simulink model "uz_ssi_interface_2023a"  (R2023a)
settings: Solver=FixedStepDiscrete  StartTime=0.0  StopTime=0.003  RelTol=1e-3
values from neighbouring files (symbols this model uses):
  binary_or_gray = false    [uz_ssi_interface_init.m]
  bit_sum = ssi_encoder_bit_width_multi_turn+ssi_encoder_bit_width_single_turn+ssi_encoder_number_of_status_bits    [uz_ssi_interface_init.m]
  delay_first_clk_on_off = true    [uz_ssi_interface_init.m]
  f_ADC = 10e3    (= 10000)    [uz_ssi_interface_init.m]
  f_clock = 100e6    (= 100000000)    [uz_ssi_interface_init.m]
  ssi_clk_divider = 25    [uz_ssi_interface_init.m]
  ssi_encoder_bit_width_multi_turn = uint32(0)    [uz_ssi_interface_init.m]
  ssi_encoder_bit_width_single_turn = uint32(14)    [uz_ssi_interface_init.m]
  ssi_encoder_number_of_status_bits = uint32(0)    [uz_ssi_interface_init.m]
  t_ADC = 1/f_ADC    (= 0.0001)    [uz_ssi_interface_init.m]
  t_clock = 1/f_clock    (= 1e-08)    [uz_ssi_interface_init.m]
undefined symbols (not defined in the file or in its folder): PLL
libraries: hdlsllib x42, simulink x14, simulink_extras x5, spsSampleandHoldLib x1
(part 2 of 2)

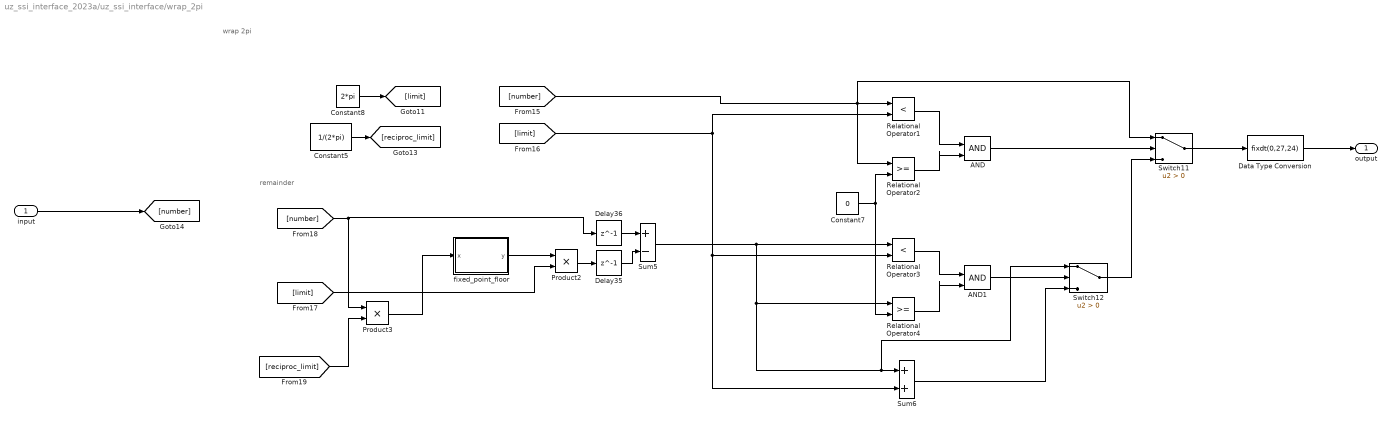
== system uz_ssi_interface_2023a/uz_ssi_interface/wrap_2pi ==
  note: wrap 2pi
  note: remainder
  input : Inport
  AND : Logic  IconShape=distinctive  AllPortsSameDT=off  OutDataTypeStr=boolean
  AND1 : Logic  IconShape=distinctive  AllPortsSameDT=off  OutDataTypeStr=boolean
  Constant5 : Constant  Value=1/(2*pi)  OutDataTypeStr=fixdt(0,18,20)  SampleTime=-1
  Constant7 : Constant  Value=0  OutDataTypeStr=fixdt(0,27,24)  SampleTime=-1
  Constant8 : Constant  Value=2*pi  OutDataTypeStr=fixdt(0,18,15)  SampleTime=-1
  Data Type Conversion : DataTypeConversion  OutDataTypeStr=fixdt(0,27,24)  SaturateOnIntegerOverflow=off  RndMeth=Floor
  Delay35 : Delay  DelayLength=1  InitialCondition=0
  Delay36 : Delay  DelayLength=1  InitialCondition=0
  Product2 : Product  OutDataTypeStr=fixdt(0,27,24)
  Product3 : Product  OutDataTypeStr=fixdt(0,27,24)
  Relational Operator1 : RelationalOperator  Operator=<  OutDataTypeStr=boolean  RndMeth=Simplest  InputSameDT=off
  Relational Operator2 : RelationalOperator  OutDataTypeStr=boolean  RndMeth=Simplest  InputSameDT=off
  Relational Operator3 : RelationalOperator  Operator=<  OutDataTypeStr=boolean  RndMeth=Simplest  InputSameDT=off
  Relational Operator4 : RelationalOperator  OutDataTypeStr=boolean  RndMeth=Simplest  InputSameDT=off
  Sum5 : Sum  Inputs=+-  OutDataTypeStr=fixdt(0,27,24)
  Sum6 : Sum  OutDataTypeStr=fixdt(0,27,24)
  Switch11 : Switch  Criteria=u2 > Threshold  SaturateOnIntegerOverflow=off  InputSameDT=off
  Switch12 : Switch  Criteria=u2 > Threshold  SaturateOnIntegerOverflow=off  InputSameDT=off
  fixed_point_floor : MATLAB Function  TreatAsAtomicUnit=on
  output : Outport
  wires:
  [number] -> Relational Operator2/1, Switch11/1, Relational Operator1/1
  Product2/1 -> Delay35/1
  [number] -> Delay36/1, Product3/1
  [reciproc_limit] -> Product3/2
  Delay35/1 -> Sum5/2
  Switch11/1 -> Data Type Conversion/1
  Relational Operator2/1 -> AND/2
  AND/1 -> Switch11/2
  Sum5/1 -> Switch12/1, Sum6/1, Relational Operator4/1, Relational Operator3/1
  Relational Operator1/1 -> AND/1
  [limit] -> Relational Operator1/2, Sum6/2, Relational Operator3/2
  Sum6/1 -> Switch12/3
  Delay36/1 -> Sum5/1
  Constant7/1 -> Relational Operator2/2, Relational Operator4/2
  Constant5/1 -> [reciproc_limit]
  Relational Operator4/1 -> AND1/2
  fixed_point_floor/1(y) -> Product2/1
  Product3/1 -> fixed_point_floor/1(x)
  AND1/1 -> Switch12/2
  [limit] -> Product2/2
  input/1 -> [number]
  Relational Operator3/1 -> AND1/1
  Switch12/1 -> Switch11/3
  Constant8/1 -> [limit]
  Data Type Conversion/1 -> output/1

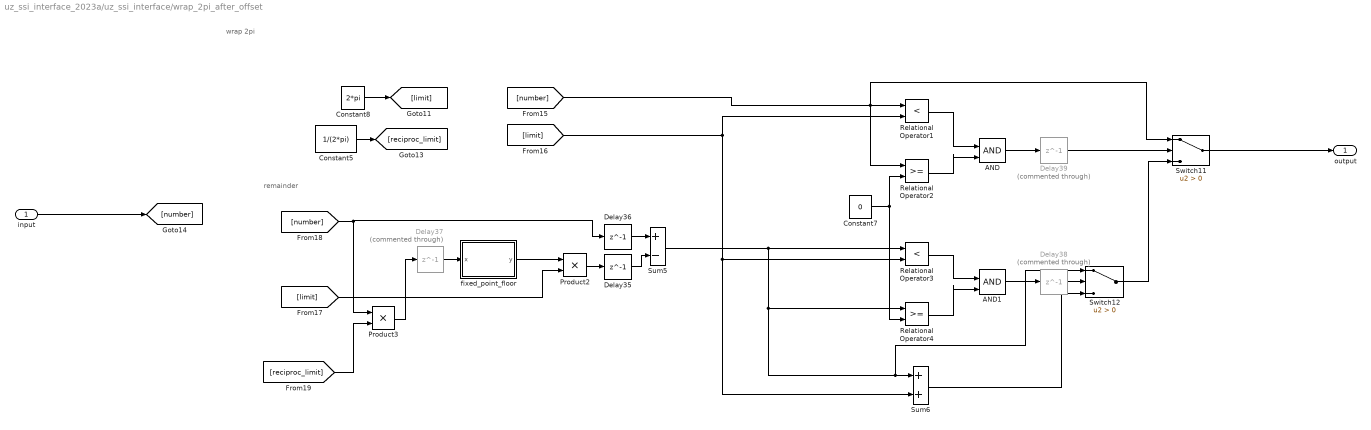
== system uz_ssi_interface_2023a/uz_ssi_interface/wrap_2pi_after_offset ==
  note: wrap 2pi
  note: remainder
  input : Inport
  AND : Logic  IconShape=distinctive  AllPortsSameDT=off  OutDataTypeStr=boolean
  AND1 : Logic  IconShape=distinctive  AllPortsSameDT=off  OutDataTypeStr=boolean
  Constant5 : Constant  Value=1/(2*pi)  OutDataTypeStr=fixdt(0,18,20)  SampleTime=-1
  Constant7 : Constant  Value=0  OutDataTypeStr=fixdt(0,27,24)  SampleTime=-1
  Constant8 : Constant  Value=2*pi  OutDataTypeStr=fixdt(0,18,15)  SampleTime=-1
  Delay35 : Delay  DelayLength=1  InitialCondition=0
  Delay36 : Delay  DelayLength=1  InitialCondition=0
  Delay37 : Delay  Commented=through  DelayLength=1  InitialCondition=0
  Delay38 : Delay  Commented=through  DelayLength=1
  Delay39 : Delay  Commented=through  DelayLength=1
  Product2 : Product  OutDataTypeStr=fixdt(0,27,24)
  Product3 : Product  OutDataTypeStr=fixdt(1,27,23)
  Relational Operator1 : RelationalOperator  Operator=<  OutDataTypeStr=boolean  RndMeth=Simplest  InputSameDT=off
  Relational Operator2 : RelationalOperator  OutDataTypeStr=boolean  RndMeth=Simplest  InputSameDT=off
  Relational Operator3 : RelationalOperator  Operator=<  OutDataTypeStr=boolean  RndMeth=Simplest  InputSameDT=off
  Relational Operator4 : RelationalOperator  OutDataTypeStr=boolean  RndMeth=Simplest  InputSameDT=off
  Sum5 : Sum  Inputs=+-  OutDataTypeStr=fixdt(0,27,24)
  Sum6 : Sum  OutDataTypeStr=fixdt(0,27,24)
  Switch11 : Switch  Criteria=u2 > Threshold  SaturateOnIntegerOverflow=off  InputSameDT=off
  Switch12 : Switch  Criteria=u2 > Threshold  SaturateOnIntegerOverflow=off  InputSameDT=off
  fixed_point_floor : MATLAB Function  TreatAsAtomicUnit=on
  output : Outport
  wires:
  [number] -> Relational Operator2/1, Switch11/1, Relational Operator1/1
  Product2/1 -> Delay35/1
  [number] -> Delay36/1, Product3/1
  [reciproc_limit] -> Product3/2
  Product3/1 -> Delay37/1
  Delay35/1 -> Sum5/2
  Switch11/1 -> output/1
  Relational Operator2/1 -> AND/2
  AND1/1 -> Delay38/1
  Delay39/1 -> Switch11/2
  Sum5/1 -> Switch12/1, Sum6/1, Relational Operator4/1, Relational Operator3/1
  Relational Operator1/1 -> AND/1
  [limit] -> Relational Operator1/2, Sum6/2, Relational Operator3/2
  AND/1 -> Delay39/1
  Sum6/1 -> Switch12/3
  Delay36/1 -> Sum5/1
  Constant7/1 -> Relational Operator2/2, Relational Operator4/2
  Constant5/1 -> [reciproc_limit]
  Relational Operator4/1 -> AND1/2
  fixed_point_floor/1(y) -> Product2/1
  Delay37/1 -> fixed_point_floor/1(x)
  Delay38/1 -> Switch12/2
  [limit] -> Product2/2
  input/1 -> [number]
  Relational Operator3/1 -> AND1/1
  Switch12/1 -> Switch11/3
  Constant8/1 -> [limit]

== matlab function uz_ssi_interface_2023a/uz_ssi_interface/sample_serial_ssi_data/sample_serial_data ==
  data: clk input; data_out output; data_in input; bit_width input; data_valid output
function [data_out, data_valid]  = sample_serial_data(clk, data_in, bit_width)
    % Function to sample serial data bits of configurable length
    % Inputs:
    %   - data_in: Single bit of serial data to be sampled (1 or 0)
    %   - clk: Input clock signal (high when data is to be sampled)
    %   - bit_width: Number of bits to be sampled (configurable length)
    %
    % Output:
    %   - data_out: Integer value of the concatenated data bits after sampling
    %   - data_valid: high when all bits have been sampled

    persistent data_buffer bit_count

    if isempty(data_buffer)
        % Initialize buffer as a fixed-point number with 64 bits and unsigned
        data_buffer = fi(0,0,64,0); 
        bit_count = uint32(bit_width); 
    end

    % Sample the data when the clock is high
    if clk == 1

        % Add the incoming bit to the data buffer
        data_buffer = bitset(data_buffer,bit_count,data_in);

        % Decrement the bit counter
        bit_count = bit_count - 1;
    end

    % When the required length is reached, output the data
    if bit_count == 0
        data_out = uint64(data_buffer);  % Convert fixed-point to uint64
        data_valid = true;
        % Reset the buffer and bit counter for the next sample
        data_buffer = fi(0,0,64,0);  % Reset buffer
        bit_count = bit_width;                   % Reset bit count
    else
        data_out = uint64(0);  % No output until the required number of bits are sampled
        data_valid = false;
    end
end

== matlab function uz_ssi_interface_2023a/uz_ssi_interface/wrap_2pi/fixed_point_floor ==
  data: x input; y output
function y = fcn(x)
%#codegen
x_floor = bitsra(x, x.FractionLength);  % Shift right to remove fraction
x_floor = bitsll(x_floor, x.FractionLength);  % Shift left to restore scale

y = x_floor;

== matlab function uz_ssi_interface_2023a/uz_ssi_interface/position_to_speed_pll/fixed_point_floor ==
  data: x input; y output
function y = fcn(x)
%#codegen
x_floor = bitsra(x, x.FractionLength);  % Shift right to remove fraction
x_floor = bitsll(x_floor, x.FractionLength);  % Shift left to restore scale

y = x_floor;

== matlab function uz_ssi_interface_2023a/uz_ssi_interface/wrap_2pi_after_offset/fixed_point_floor ==
  data: x input; y output
function y = fcn(x)
%#codegen
x_floor = bitsra(x, x.FractionLength);  % Shift right to remove fraction
x_floor = bitsll(x_floor, x.FractionLength);  % Shift left to restore scale

y = x_floor;

== matlab function uz_ssi_interface_2023a/uz_ssi_interface/sample_serial_ssi_data/slice_position_and_status ==
  data: data input; bit_width_mt input; pos_raw_st output; bit_width_st input; bit_width_status input; pos_raw_mt output; raw_status output; shift_val_mt input; shift_val_st input
function [pos_raw_st, pos_raw_mt, raw_status] = slice_pos_and_status(data, bit_width_mt, bit_width_st, bit_width_status, shift_val_mt, shift_val_st)

    % Extract pos_raw_mt (from MSB), then right-align into uint32
    shifted_mt = bitshift(data, -shift_val_mt);
    mask_mt = uint64(2^bit_width_mt-1);
    pos_raw_mt = uint32(bitand(shifted_mt, mask_mt));

    % Extract pos_raw_st (middle field), then right-align into uint32
    shifted_st = bitshift(data, -shift_val_st);
    mask_st = uint64(2^bit_width_st-1);
    pos_raw_st = uint32(bitand(shifted_st, mask_st));

    % Extract raw_status (LSBs already), right-align into uint32
    mask_status = uint64(2^(uint32(bit_width_status))-1);
    raw_status = uint32(bitand(data,mask_status));
end

== matlab function uz_ssi_interface_2023a/ssi_encoder/MATLAB Function ==
  data: u input; y output
function y = BinaryToGray(u)
%#codegen

y = bitxor(u,(bitshift(u,-1)));

== matlab function uz_ssi_interface_2023a/uz_ssi_interface/Gray_code_to_binary/gray_to_bin_st ==
  data: gray input; binary output
function binary  = GrayToBinary(gray)
%#codegen

binary = gray;
    for i = 1:24 % 24 shifts for 25-bit word
        shift_val = bitshift(gray, -i);
        binary = bitxor(binary, shift_val);
    end
end

== matlab function uz_ssi_interface_2023a/uz_ssi_interface/Gray_code_to_binary/gray_to_bin_mt ==
  data: gray input; binary output
function binary  = GrayToBinary(gray)
%#codegen

binary = gray;
    for i = 1:24 % 24 shifts for 25-bit word
        shift_val = bitshift(gray, -i);
        binary = bitxor(binary, shift_val);
    end
end
